simulink model "fuzzycontroller3012"  (R2018b)
settings: Solver=VariableStepAuto  StartTime=0.0  StopTime=10.0  RelTol=1e-3
libraries: fuzblock x1
settings Model: Creator=student  LastModifiedBy=student

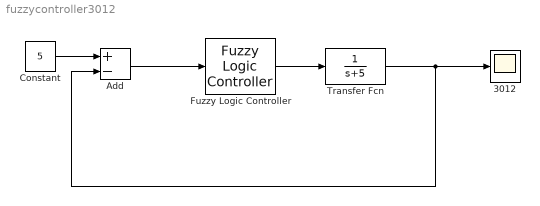
== system fuzzycontroller3012 ==
  3012 : Scope
  Add : Sum  Inputs=+-
  Constant : Constant  Value=5
  Fuzzy Logic Controller : fuzblock/Fuzzy Logic  Controller  FIS='fuzzycontroller3012.fis'  OutputSampleNumber=101  DataType=double  FuzzifiedInputs=off  RuleFiringStrengths=off  RuleOutputs=off  AggregatedOutputs=off  SimulateUsing=Interpreted execution  OutOfRangeInputValueMessage=warning  NoRuleFiredMessage=warning  EmptyOutputFuzzySetMessage=warning
  Transfer Fcn : TransferFcn  Denominator=[1 5]
  wires:
  Constant/1 -> Add/1
  Fuzzy Logic Controller/1 -> Transfer Fcn/1
  Add/1 -> Fuzzy Logic Controller/1
  Transfer Fcn/1 -> Add/2, 3012/1
